simulink model "czasowe"  (R2022b)
settings: Solver=VariableStepAuto  StartTime=0.0  StopTime=100  RelTol=1e-3
settings Model: Creator=zuzanna  LastModifiedBy=zuzanna

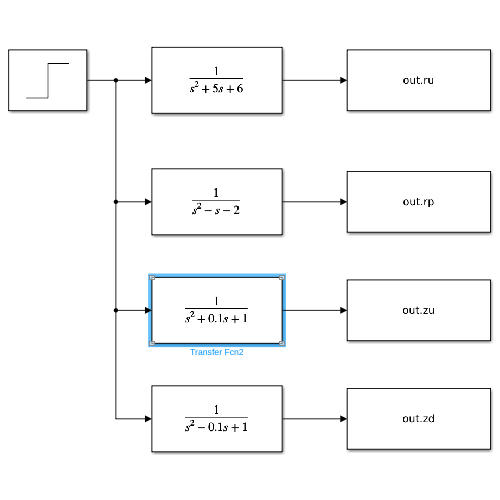
[thumbnail: Simulink's stored preview of the top-level diagram]
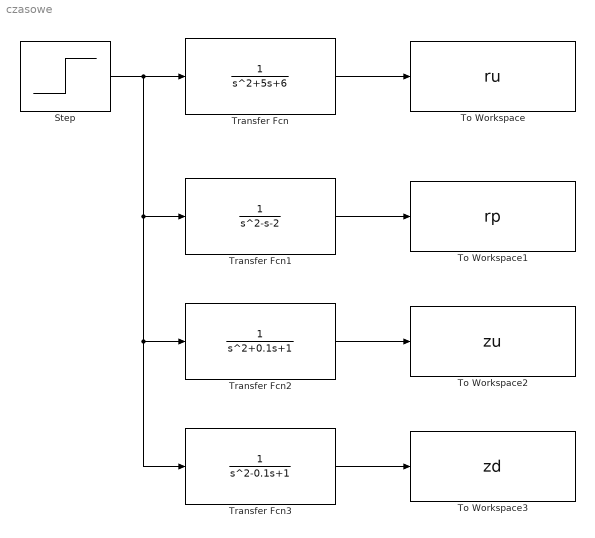
== system czasowe ==
  Step : Step  Time=0  SampleTime=0
  To Workspace : ToWorkspace  VariableName=ru  SampleTime=-1
  To Workspace1 : ToWorkspace  VariableName=rp  SampleTime=-1
  To Workspace2 : ToWorkspace  VariableName=zu  SampleTime=-1
  To Workspace3 : ToWorkspace  VariableName=zd  SampleTime=-1
  Transfer Fcn : TransferFcn  Denominator=[1 5 6]
  Transfer Fcn1 : TransferFcn  Denominator=[1 -1 -2]
  Transfer Fcn2 : TransferFcn  Denominator=[1 0.1 1]
  Transfer Fcn3 : TransferFcn  Denominator=[1 -0.1 1]
  wires:
  Step/1 -> Transfer Fcn3/1, Transfer Fcn2/1, Transfer Fcn1/1, Transfer Fcn/1
  Transfer Fcn/1 -> To Workspace/1
  Transfer Fcn1/1 -> To Workspace1/1
  Transfer Fcn2/1 -> To Workspace2/1
  Transfer Fcn3/1 -> To Workspace3/1
